simulink model "LS1_3_clrd"  (R2024a)
settings: Solver=FixedStepAuto  StartTime=0.0  StopTime=1000  FixedStep=0.3  RelTol=1e-3
libraries: dspsrcs4 x2
settings Model: Creator=mergenelos  LastModifiedBy=mergenelos

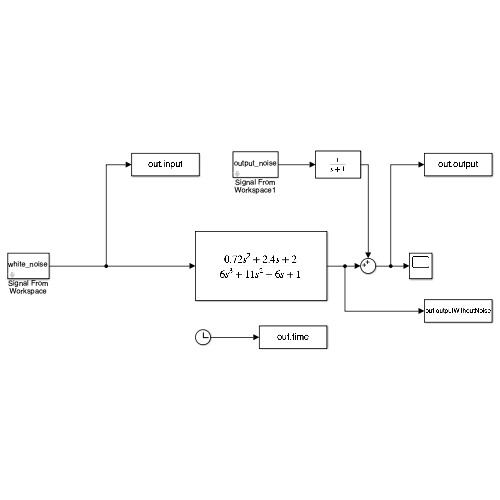
[thumbnail: Simulink's stored preview of the top-level diagram]
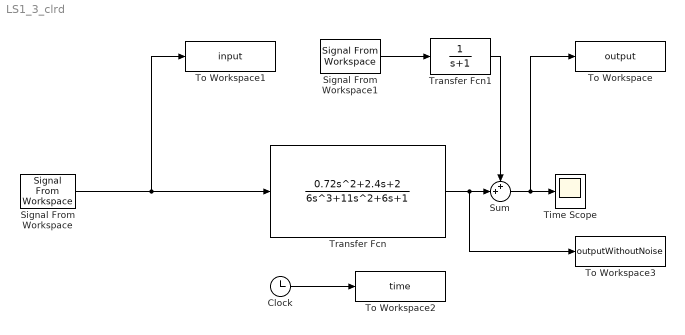
== system LS1_3_clrd ==
  Clock : Clock
  Signal From Workspace : dspsrcs4/Signal From Workspace  X=white_noise  Ts=0.3  nsamps=1  OutputAfterFinalValue=Setting to zero  ignoreOrWarnInputAndFrameLengths=off  OutputFrames=off
  Signal From Workspace1 : dspsrcs4/Signal From Workspace  X=output_noise  Ts=0.3  nsamps=1  OutputAfterFinalValue=Setting to zero  ignoreOrWarnInputAndFrameLengths=off  OutputFrames=off
  Sum : Sum  Inputs=++|
  Time Scope : Scope
  To Workspace : ToWorkspace  VariableName=output  SaveFormat=Timeseries  SampleTime=-1
  To Workspace1 : ToWorkspace  VariableName=input  SaveFormat=Timeseries  SampleTime=-1
  To Workspace2 : ToWorkspace  VariableName=time  SaveFormat=Timeseries  SampleTime=-1
  To Workspace3 : ToWorkspace  VariableName=outputWithoutNoise  SaveFormat=Timeseries  SampleTime=-1
  Transfer Fcn : TransferFcn  Numerator=[0.72 2.4 2]  Denominator=[6 11 6 1]
  Transfer Fcn1 : TransferFcn  Denominator=[1 1]
  wires:
  Signal From Workspace/1 -> To Workspace1/1, Transfer Fcn/1
  Clock/1 -> To Workspace2/1
  Sum/1 -> To Workspace/1, Time Scope/1
  Signal From Workspace1/1 -> Transfer Fcn1/1
  Transfer Fcn/1 -> To Workspace3/1, Sum/2
  Transfer Fcn1/1 -> Sum/1
